simulink model "model"  (R2020b)
settings: Solver=ode4  StartTime=0.0  StopTime=200  FixedStep=0.1  RelTol=1e-3
values from neighbouring files (symbols this model uses):
  b = 50    [parameters.m]
  k_one = 50    [parameters.m]
  k_two = 10    [parameters.m]
  m_one = 100    [parameters.m]
  m_two = 20    [parameters.m]
settings Model: Creator=Pavan  LastModifiedBy=Pavan

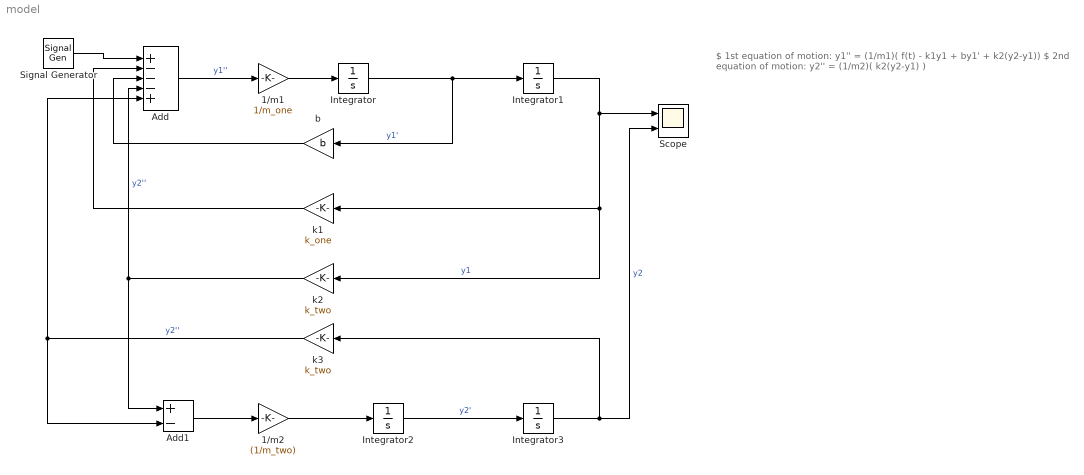
== system model ==
  note: $ 1st equation of motion:
      | y1'' = (1/m1)( f(t) - k1y1 + by1' + k2(y2-y1))
      |
      | $ 2nd equation of motion:
      | y2'' = (1/m2)( k2(y2-y1) )
  1/m1 : Gain  Gain=1/m_one
  1/m2 : Gain  Gain=(1/m_two)
  Add : Sum  Inputs=+---+
  Add1 : Sum  Inputs=+-
  Integrator{,1..3} (4 alike) : Integrator
  Scope : Scope  NumInputPorts=2
  Signal Generator : SignalGenerator  Amplitude=2  Frequency=0.7071  Units=rad/sec
  b : Gain  Gain=b
  k1 : Gain  Gain=k_one
  k2 : Gain  Gain=k_two
  k3 : Gain  Gain=k_two
  wires:
  Integrator/1 -> b/1, Integrator1/1  "y1'"
  Integrator2/1 -> Integrator3/1  "y2'"
  Add/1 -> 1/m1/1  "y1''"
  Integrator1/1 -> k2/1, k1/1, Scope/1  "y1"
  k2/1 -> Add1/1, Add/4  "y2''"
  1/m1/1 -> Integrator/1
  b/1 -> Add/3
  Signal Generator/1 -> Add/1
  k1/1 -> Add/2
  Integrator3/1 -> k3/1, Scope/2  "y2"
  1/m2/1 -> Integrator2/1
  Add1/1 -> 1/m2/1
  k3/1 -> Add1/2, Add/5  "y2''"
